simulink model "FuelSimModel"  (R2022a)
settings: Solver=ode1  StartTime=0.0  StopTime=40  FixedStep=0.01  RelTol=1e-3  EnableMultiTasking=on
StopFcn:
  | FuelControlAutoGrading
undefined symbols (not defined in the file or in its folder): AFs, eta, KM, N, R, T, tau, tauM, TL, Vd, Vi, X
libraries: simulink x1
settings Model: Creator=burl  LastModifiedBy=Chaitanya
settings SolverCC: AlgebraicLoopSolver=TrustRegion
settings DataIOCC: LimitDataPoints=on  SaveFormat=Array  ReturnWorkspaceOutputs=off
settings OptimizationCC: BlockReduction=off  OptimizeBlockIOStorage=off  BufferReuse=off  GlobalBufferReuse=off  ExpressionFolding=off  LocalBlockOutputs=off  LifeSpan=inf  OptimizeDataStoreBuffers=off  BusAssignmentInplaceUpdate=off
settings DebuggingCC: UnderspecifiedInitializationDetection=Classic  MergeDetectMultiDrivingBlocksExec=none  SolverPrmCheckMsg=warning  UnconnectedInputMsg=warning  UnconnectedOutputMsg=warning  UnconnectedLineMsg=warning  StateNameClashWarn=warning  SFUnexpectedBacktrackingDiag=warning  SFNoUnconditionalDefaultTransitionDiag=warning  SFExecutionAtInitializationDiag=none  SFMachineParentedDataDiag=warning  ArithmeticOperatorsInVariantConditions=warning
settings HardwareCC: ProdBitPerPointer=32  ProdBitPerSizeT=32  ProdBitPerPtrDiffT=32  ProdLargestAtomicFloat=None  ProdWordSize=32  ProdHWDeviceType=Generic->Custom  TargetIntDivRoundTo=Zero  TargetEndianess=LittleEndian  TargetHWDeviceType=Generic->Custom
settings ModelReferenceCC: PropagateSignalLabelsOutOfModel=off
settings SFSimCC: SimUseLocalCustomCode=off  CustomCodeUndefinedFunction=UseInterfaceOnly
settings RTWCC: Description=dSPACE DS1006 Hardware Platform  SystemTargetFile=rti1006.tlc  MakeCommand=make_rti  TemplateMakefile=rti1006.tmf  RTWUseLocalCustomCode=off
settings CodeAppCC: StateflowObjectComments=on
settings STFCustomTargetCC: ParMdlRefBuildCompliant=on  MatFileLogging=on  CPPClassGenCompliant=on  SystemTargetFile=rti1006.tlc
settings GRTTargetCC: TargetLangStandard=C89/C90 (ANSI)  CompOptLevelCompliant=off  ConcurrentExecutionCompliant=off  CombineOutputUpdateFcns=off  GRTInterface=on  UseToolchainInfoCompliant=off
settings ConfigComp: CovMetricSettings=dw  CovSaveCumulativeToWorkspaceVar=on  CovSaveSingleToWorkspaceVar=on  CovExternalEMLEnable=off

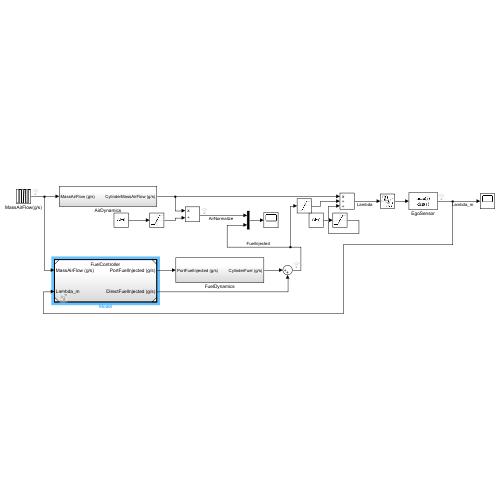
[thumbnail: Simulink's stored preview of the top-level diagram]
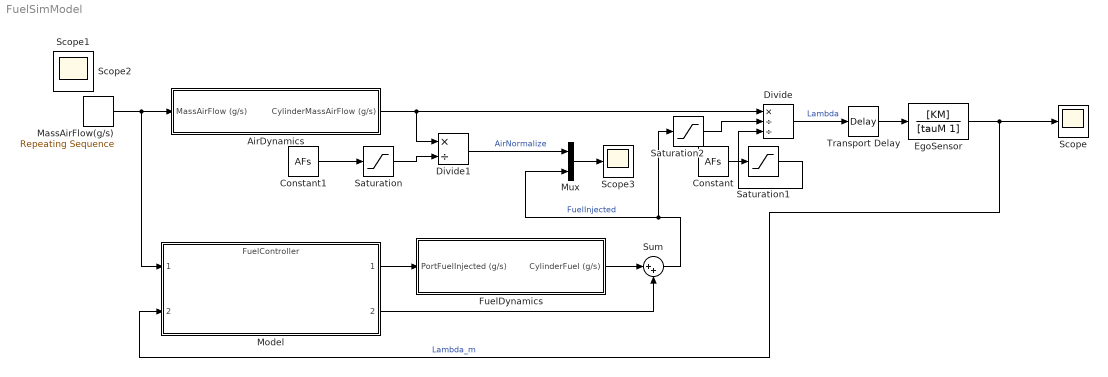
== system FuelSimModel ==
  AirDynamics : Subsystem
  Constant : Constant  Value=AFs
  Constant1 : Constant  Value=AFs
  Divide : Product  Inputs=*//
  Divide1 : Product  Inputs=*/
  EgoSensor : TransferFcn  Numerator=[KM]  Denominator=[tauM 1]
  FuelDynamics : Subsystem
  MassAirFlow(g/s) : simulink/Sources/Repeating Sequence  rep_seq_t=[0 10 10.1 20 20.1]  rep_seq_y=[10 10 20 20 10]
  Model : ModelReference  ModelNameDialog=FuelController.slx  SimulationMode=Normal  ModelReferenceVersion=9.8
  Mux : Mux  Inputs=2
  Saturation : Saturate  UpperLimit=10000000  LowerLimit=0.0005
  Saturation1 : Saturate  UpperLimit=10000000  LowerLimit=0.0005
  Saturation2 : Saturate  UpperLimit=10000000  LowerLimit=0.0005
  Scope{,1..3} (4 alike) : Scope
  Sum : Sum  Inputs=|++
  Transport Delay : TransportDelay  DelayTime=TL
  wires:
  Divide/1 -> Transport Delay/1  "Lambda"
  MassAirFlow(g/s)/1 -> Model/1, AirDynamics/1(MassAirFlow (g/s))
  Model/1 -> FuelDynamics/1(PortFuelInjected (g/s))
  EgoSensor/1 -> Model/2, Scope/1  "Lambda_m"
  Transport Delay/1 -> EgoSensor/1
  AirDynamics/1(CylinderMassAirFlow (g/s)) -> Divide1/1, Divide/1
  FuelDynamics/1(CylinderFuel (g/s)) -> Sum/1
  Mux/1 -> Scope3/1
  Divide1/1 -> Mux/1  "AirNormalize"
  Sum/1 -> Saturation2/1, Mux/2  "FuelInjected"
  Model/2 -> Sum/2
  Constant1/1 -> Saturation/1
  Saturation/1 -> Divide1/2
  Constant/1 -> Saturation1/1
  Saturation1/1 -> Divide/3
  Saturation2/1 -> Divide/2

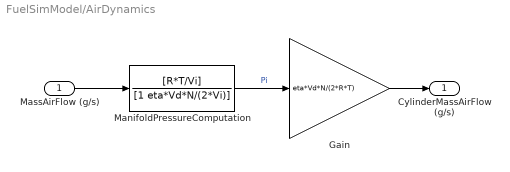
== system FuelSimModel/AirDynamics ==
  MassAirFlow (g/s) : Inport
  Gain : Gain  Gain=eta*Vd*N/(2*R*T)
  ManifoldPressureComputation : TransferFcn  Numerator=[R*T/Vi]  Denominator=[1 eta*Vd*N/(2*Vi)]
  CylinderMassAirFlow (g/s) : Outport  VectorParamsAs1DForOutWhenUnconnected=off
  wires:
  MassAirFlow (g/s)/1 -> ManifoldPressureComputation/1
  ManifoldPressureComputation/1 -> Gain/1  "Pi"
  Gain/1 -> CylinderMassAirFlow (g/s)/1

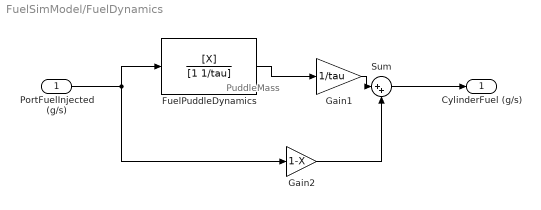
== system FuelSimModel/FuelDynamics ==
  note: PuddleMass
  PortFuelInjected (g/s) : Inport
  FuelPuddleDynamics : TransferFcn  Numerator=[X]  Denominator=[1 1/tau]
  Gain1 : Gain  Gain=1/tau
  Gain2 : Gain  Gain=1-X
  Sum : Sum  Inputs=|++
  CylinderFuel (g/s) : Outport  VectorParamsAs1DForOutWhenUnconnected=off
  wires:
  PortFuelInjected (g/s)/1 -> Gain2/1, FuelPuddleDynamics/1
  FuelPuddleDynamics/1 -> Gain1/1
  Gain1/1 -> Sum/1
  Gain2/1 -> Sum/2
  Sum/1 -> CylinderFuel (g/s)/1
